simulink model "msd"  (R2022b)
settings: Solver=VariableStepAuto  StartTime=0.0  StopTime=50  RelTol=1e-6
settings Model: Creator=Rocksmithed  LastModifiedBy=86156
settings SolverCC: AlgebraicLoopSolver=TrustRegion
settings DataIOCC: SaveFormat=Array
settings DebuggingCC: UnconnectedInputMsg=warning  UnconnectedOutputMsg=warning  UnconnectedLineMsg=warning  SFMachineParentedDataDiag=warning
settings ModelReferenceCC: EnableRefExpFcnMdlSchedulingChecks=on

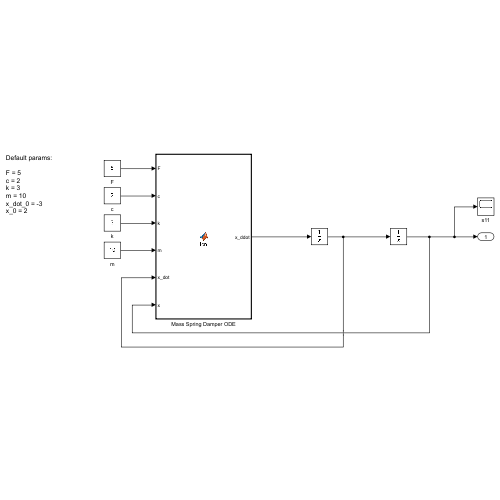
[thumbnail: Simulink's stored preview of the top-level diagram]
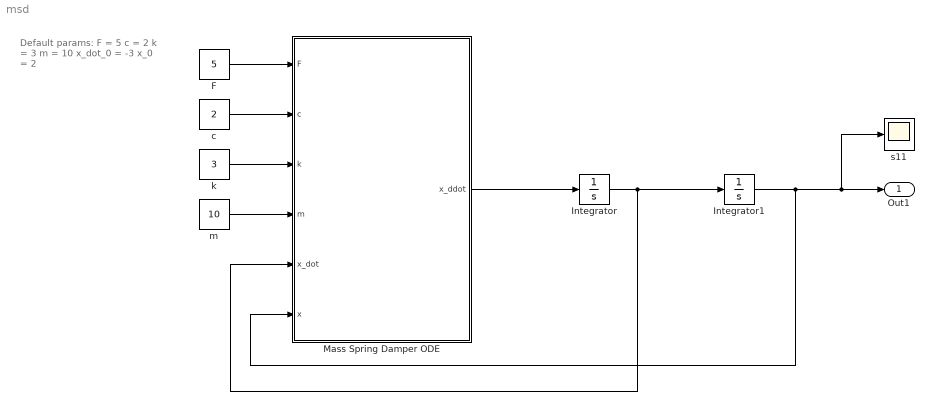
== system msd ==
  note: Default params:
      |
      | F = 5
      | c = 2
      | k = 3
      | m = 10
      | x_dot_0 = -3
      | x_0 = 2
  F : Constant  Value=5
  Integrator : Integrator  InitialCondition=-3
  Integrator1 : Integrator  InitialCondition=2
  Mass Spring Damper ODE : MATLAB Function  TreatAsAtomicUnit=on
  c : Constant  Value=2
  k : Constant  Value=3
  m : Constant  Value=10
  s11 : Scope
  Out1 : Outport
  wires:
  F/1 -> Mass Spring Damper ODE/1(F)
  c/1 -> Mass Spring Damper ODE/2(c)
  k/1 -> Mass Spring Damper ODE/3(k)
  m/1 -> Mass Spring Damper ODE/4(m)
  Integrator/1 -> Mass Spring Damper ODE/5(x_dot), Integrator1/1
  Integrator1/1 -> Mass Spring Damper ODE/6(x), s11/1, Out1/1
  Mass Spring Damper ODE/1(x_ddot) -> Integrator/1

== matlab function msd/Mass Spring Damper ODE ==
  data: F input; x_ddot output; c input; k input; m input; x_dot input; x input
function x_ddot = fcn(F,c,k,m,x_dot,x)

   % Write your expression for x_ddot here in terms of the inputs
   x_ddot = -(-F+c.*x_dot+k.*x)./m;
end
